simulink subsystem "NavigationSolution"  (R2021a)
settings: Solver=VariableStepAuto  StartTime=0.0  StopTime=10.0  RelTol=1e-3
settings Model: Creator=Laura  LastModifiedBy=Laura

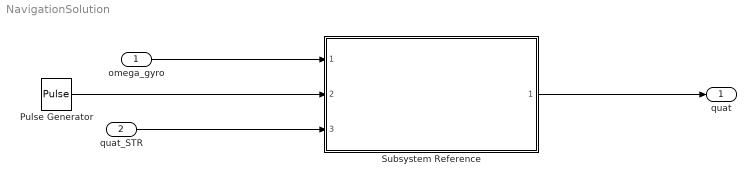
== system NavigationSolution ==
  omega_gyro : Inport
  quat_STR : Inport  Port=2
  Pulse Generator : DiscretePulseGenerator  PulseType=Time based  Period=1/10  PulseWidth=5
  Subsystem Reference : Subsystem  ReferencedSubsystem=GyroStarTrackerReset
  quat : Outport
  wires:
  Pulse Generator/1 -> Subsystem Reference/2
  omega_gyro/1 -> Subsystem Reference/1
  quat_STR/1 -> Subsystem Reference/3
  Subsystem Reference/1 -> quat/1
